simulink model "graph3"  (R2021b)
settings: Solver=VariableStepAuto  StartTime=0.0  StopTime=10.0  RelTol=1e-3
settings Model: Creator=hamza  LastModifiedBy=hamza

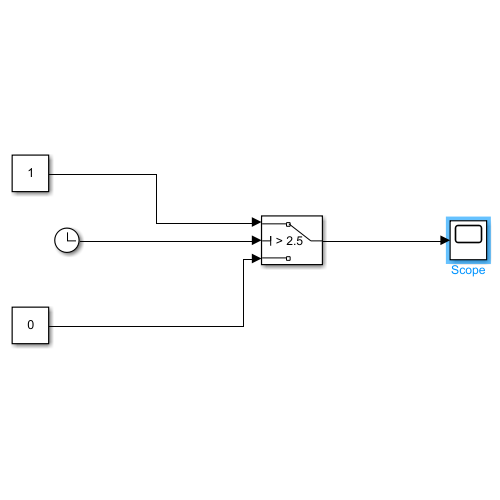
[thumbnail: Simulink's stored preview of the top-level diagram]
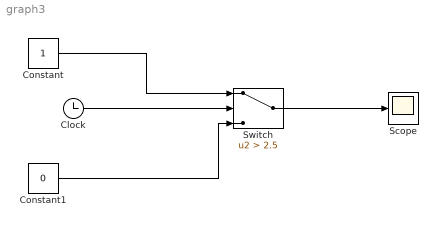
== system graph3 ==
  Clock : Clock
  Constant : Constant
  Constant1 : Constant  Value=0
  Scope : Scope
  Switch : Switch  Criteria=u2 > Threshold  Threshold=2.5
  wires:
  Clock/1 -> Switch/2
  Constant1/1 -> Switch/3
  Constant/1 -> Switch/1
  Switch/1 -> Scope/1
